simulink model "testFrame_PIControler"  (R2020b)
settings: Solver=FixedStepDiscrete  StartTime=0.0  StopTime=10.0  FixedStep=2e-4  RelTol=1e-3
undefined symbols (not defined in the file): BrkPoints, Down, Ki_dAxis, Ki_qAxis, Kp_dAxis, Kp_qAxis, pwmTableData, Ts, Up
libraries: eePwmGenerator x3, mcbcontrolslib x2
settings Model: DataDictionary=MotorControl.sldd  Creator=unix  LastModifiedBy=unix
settings DebuggingCC: SignalRangeChecking=error  IntegerOverflowMsg=error  ParameterUnderflowMsg=error  IntegerSaturationMsg=error

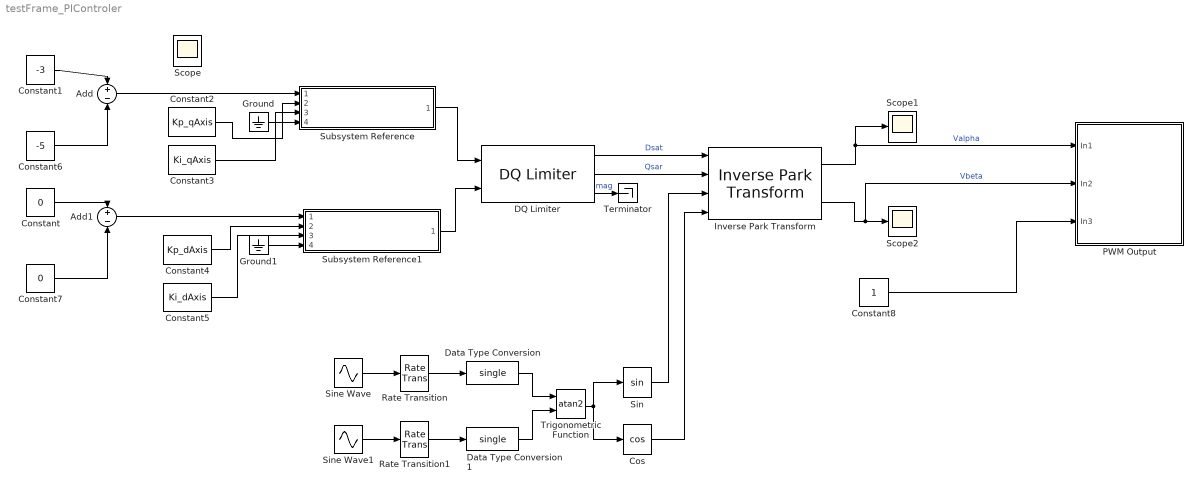
== system testFrame_PIControler ==
  Add : Sum  Inputs=+-
  Add1 : Sum  Inputs=+-
  Constant : Constant  Value=0  OutDataTypeStr=single
  Constant1 : Constant  Value=-3  OutDataTypeStr=single
  Constant2 : Constant  Value=Kp_qAxis  OutDataTypeStr=single
  Constant3 : Constant  Value=Ki_qAxis  OutDataTypeStr=single
  Constant4 : Constant  Value=Kp_dAxis  OutDataTypeStr=single
  Constant5 : Constant  Value=Ki_dAxis  OutDataTypeStr=single
  Constant6 : Constant  Value=-5  OutDataTypeStr=single
  Constant7 : Constant  Value=0  OutDataTypeStr=single
  Constant8 : Constant
  Cos : Trigonometry  Operator=cos
  DQ Limiter : mcbcontrolslib/DQ Limiter  Vmax=d_q_Voltage_Limiter_max
      settings: SourceProductBaseCode=MT
  Data Type Conversion : DataTypeConversion  OutDataTypeStr=single
  Data Type Conversion1 : DataTypeConversion  OutDataTypeStr=single
  Ground : Ground
  Ground1 : Ground
  Inverse Park Transform : mcbcontrolslib/Inverse Park Transform  AxisAlignment=D-axis
  PWM Output : Subsystem
  Rate Transition : RateTransition
  Rate Transition1 : RateTransition
  Scope1 : Scope
  Scope2 : Scope
  Sin : Trigonometry
  Sine Wave : Sin  Amplitude=3  Frequency=60  SampleTime=0
  Sine Wave1 : Sin  Amplitude=3  Frequency=60  Phase=pi/2  SampleTime=0
  Subsystem Reference : Subsystem  ReferencedSubsystem=PID_custom
  Subsystem Reference1 : Subsystem  ReferencedSubsystem=PID_custom
  Terminator : Terminator
  Trigonometric Function : Trigonometry  Operator=atan2
  Scope : Scope
  wires:
  Add/1 -> Subsystem Reference/1
  Add1/1 -> Subsystem Reference1/1
  Constant/1 -> Add1/1
  Constant1/1 -> Add/1
  Ground/1 -> Subsystem Reference/4
  Ground1/1 -> Subsystem Reference1/4
  Constant2/1 -> Subsystem Reference/2
  Constant3/1 -> Subsystem Reference/3
  Constant4/1 -> Subsystem Reference1/2
  Constant5/1 -> Subsystem Reference1/3
  Subsystem Reference/1 -> DQ Limiter/1
  Subsystem Reference1/1 -> DQ Limiter/2
  DQ Limiter/1 -> Inverse Park Transform/1  "Dsat"
  DQ Limiter/2 -> Inverse Park Transform/2  "Qsar"
  DQ Limiter/3 -> Terminator/1  "mag"
  Constant6/1 -> Add/2
  Constant7/1 -> Add1/2
  Sine Wave/1 -> Rate Transition/1
  Sine Wave1/1 -> Rate Transition1/1
  Rate Transition/1 -> Data Type Conversion/1
  Rate Transition1/1 -> Data Type Conversion1/1
  Data Type Conversion/1 -> Trigonometric Function/1
  Data Type Conversion1/1 -> Trigonometric Function/2
  Cos/1 -> Inverse Park Transform/4
  Trigonometric Function/1 -> Sin/1, Cos/1
  Sin/1 -> Inverse Park Transform/3
  Inverse Park Transform/2 -> PWM Output/2(In2), Scope2/1  "Vbeta"
  Inverse Park Transform/1 -> PWM Output/1(In1), Scope1/1  "Valpha"
  Constant8/1 -> PWM Output/3(In3)

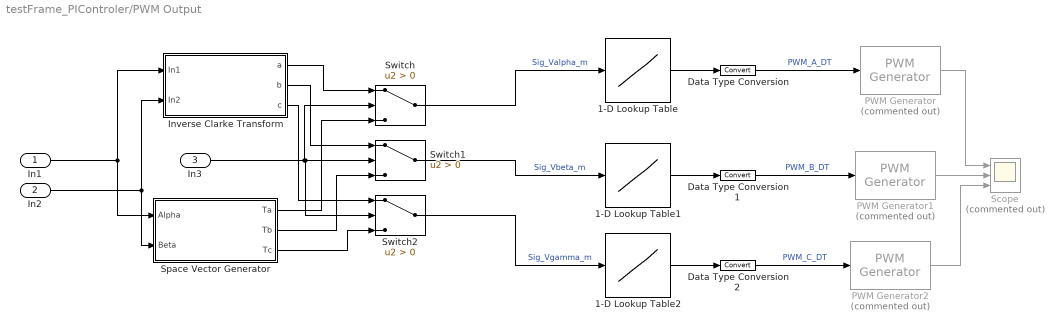
== system testFrame_PIControler/PWM Output ==
  In1 : Inport
  In2 : Inport  Port=2
  In3 : Inport  Port=3
  1-D Lookup Table : Lookup_n-D  NumberOfTableDimensions=1  BreakpointsForDimension1=BrkPoints  Table=pwmTableData  ExtrapMethod=Clip  InternalRulePriority=Speed  OutDataTypeStr=uint16  RndMeth=Simplest  SaturateOnIntegerOverflow=on  InputSameDT=on
  1-D Lookup Table1 : Lookup_n-D  NumberOfTableDimensions=1  BreakpointsForDimension1=BrkPoints  Table=pwmTableData  ExtrapMethod=Clip  InternalRulePriority=Speed  OutDataTypeStr=uint16  RndMeth=Simplest  SaturateOnIntegerOverflow=on  InputSameDT=on
  1-D Lookup Table2 : Lookup_n-D  NumberOfTableDimensions=1  BreakpointsForDimension1=BrkPoints  Table=pwmTableData  ExtrapMethod=Clip  InternalRulePriority=Speed  OutDataTypeStr=uint16  RndMeth=Simplest  SaturateOnIntegerOverflow=on  InputSameDT=on
  Data Type Conversion : DataTypeConversion
  Data Type Conversion1 : DataTypeConversion
  Data Type Conversion2 : DataTypeConversion
  Inverse Clarke Transform : Subsystem  TreatAsAtomicUnit=on  mask(Inverse Clarke Transform){}
      mask help:
      | <p>Compute Inverse Clarke transformation on balanced 2-phase orthogonal inputs into balanced 3-phase outputs.
      | <br><br>
      | The block accepts &alpha;-&beta; axis components and outputs corresponding 3-phase outputs, where phase-a axis is aligned with &alpha;-axis.</p>
      mask Help: eval('mcb.internal.helpview(''inverseclarketransform'')')
      mask Display: mcb.internal.drawIcons('invClarke',1);
  PWM Generator : eePwmGenerator/PWM Generator  Commented=on  CarrCount=Up-Down  Tper=10*Ts  Ts=Ts
  PWM Generator1 : eePwmGenerator/PWM Generator  Commented=on  CarrCount=Up-Down  Tper=10*Ts  Ts=Ts
  PWM Generator2 : eePwmGenerator/PWM Generator  Commented=on  CarrCount=Up-Down  Tper=10*Ts  Ts=Ts
  Scope : Scope  Commented=on  NumInputPorts=3
  Space Vector Generator : Subsystem  TreatAsAtomicUnit=on  mask(Space Vector Generator){}
      mask help:
      | <p>Generate space vector modulation signals from stator reference voltages described by  &alpha;-&beta; components.
      | <br><br>
      | The block accepts V<sub>&alpha;</sub> and V<sub>&beta;</sub> voltages and outputs corresponding space vector modulation voltages.</p>
      mask Help: eval('mcb.internal.helpview(''spacevectorgenerator'')')
      mask Display: mcb.internal.drawIcons('SVPWM',1);
  Switch : Switch  Criteria=u2 > Threshold
  Switch1 : Switch  Criteria=u2 > Threshold
  Switch2 : Switch  Criteria=u2 > Threshold
  wires:
  In2/1 -> Space Vector Generator/2(Beta), Inverse Clarke Transform/2(In2)
  In1/1 -> Space Vector Generator/1(Alpha), Inverse Clarke Transform/1(In1)
  Switch/1 -> 1-D Lookup Table/1  "Sig_Valpha_m"
  1-D Lookup Table/1 -> Data Type Conversion/1
  Switch1/1 -> 1-D Lookup Table1/1  "Sig_Vbeta_m"
  Switch2/1 -> 1-D Lookup Table2/1  "Sig_Vgamma_m"
  PWM Generator/1 -> Scope/1
  1-D Lookup Table2/1 -> Data Type Conversion2/1
  1-D Lookup Table1/1 -> Data Type Conversion1/1
  PWM Generator1/1 -> Scope/2
  PWM Generator2/1 -> Scope/3
  Data Type Conversion/1 -> PWM Generator/1  "PWM_A_DT"
  Data Type Conversion1/1 -> PWM Generator1/1  "PWM_B_DT"
  Data Type Conversion2/1 -> PWM Generator2/1  "PWM_C_DT"
  Space Vector Generator/1(Ta) -> Switch/3
  Space Vector Generator/2(Tb) -> Switch1/3
  Space Vector Generator/3(Tc) -> Switch2/3
  Inverse Clarke Transform/1(a) -> Switch/1
  Inverse Clarke Transform/2(b) -> Switch1/1
  Inverse Clarke Transform/3(c) -> Switch2/1
  In3/1 -> Switch2/2, Switch1/2, Switch/2

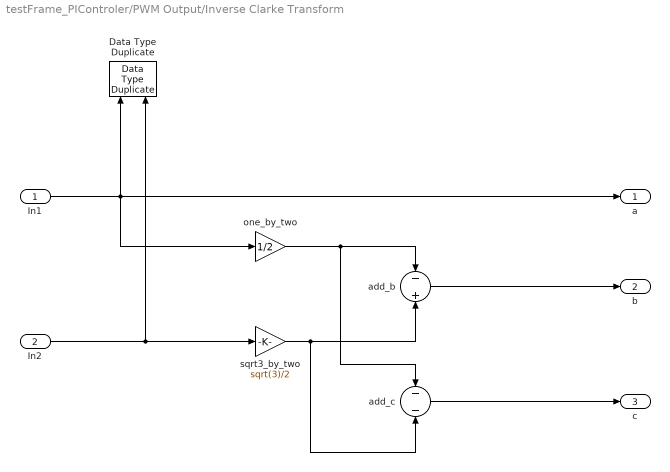
== system testFrame_PIControler/PWM Output/Inverse Clarke Transform ==
  In1 : Inport
  In2 : Inport  Port=2
  Data Type Duplicate : DataTypeDuplicate
  add_b : Sum  Inputs=-+  RndMeth=Simplest  OutDataTypeStr=Inherit: Same as first input
  add_c : Sum  Inputs=--  RndMeth=Simplest  OutDataTypeStr=Inherit: Same as first input
  one_by_two : Gain  Gain=1/2  RndMeth=Simplest  OutDataTypeStr=Inherit: Same as input
  sqrt3_by_two : Gain  Gain=sqrt(3)/2  RndMeth=Simplest  OutDataTypeStr=Inherit: Same as input
  a : Outport  VectorParamsAs1DForOutWhenUnconnected=off
  b : Outport  Port=2  VectorParamsAs1DForOutWhenUnconnected=off
  c : Outport  Port=3  VectorParamsAs1DForOutWhenUnconnected=off
  wires:
  add_c/1 -> c/1
  sqrt3_by_two/1 -> add_c/2, add_b/2
  In1/1 -> one_by_two/1, Data Type Duplicate/1, a/1
  one_by_two/1 -> add_b/1, add_c/1
  In2/1 -> sqrt3_by_two/1, Data Type Duplicate/2
  add_b/1 -> b/1

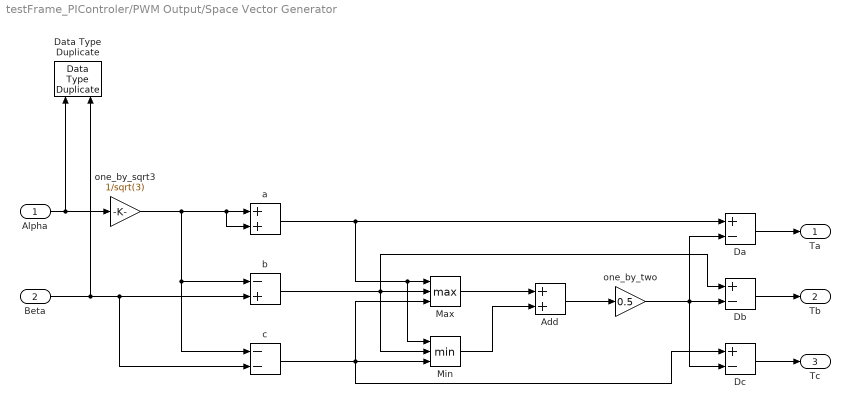
== system testFrame_PIControler/PWM Output/Space Vector Generator ==
  Alpha : Inport
  Beta : Inport  Port=2
  Add : Sum  RndMeth=Simplest  OutDataTypeStr=Inherit: Same as first input
  Da : Sum  Inputs=+-  RndMeth=Simplest  OutDataTypeStr=Inherit: Same as first input
  Data Type Duplicate : DataTypeDuplicate
  Db : Sum  Inputs=+-  RndMeth=Simplest  OutDataTypeStr=Inherit: Same as first input
  Dc : Sum  Inputs=+-  RndMeth=Simplest  OutDataTypeStr=Inherit: Same as first input
  Max : MinMax  Function=max  Inputs=3  RndMeth=Simplest
  Min : MinMax  Inputs=3  RndMeth=Simplest
  a : Sum  RndMeth=Simplest  OutDataTypeStr=Inherit: Same as first input
  b : Sum  Inputs=-+  RndMeth=Simplest  OutDataTypeStr=Inherit: Same as first input
  c : Sum  Inputs=--  RndMeth=Simplest  OutDataTypeStr=Inherit: Same as first input
  one_by_sqrt3 : Gain  Gain=1/sqrt(3)  RndMeth=Simplest  OutDataTypeStr=Inherit: Same as input  ParamDataTypeStr=Inherit: Same as input
  one_by_two : Gain  Gain=0.5  RndMeth=Simplest  OutDataTypeStr=Inherit: Same as input  ParamDataTypeStr=Inherit: Same as input
  Ta : Outport  VectorParamsAs1DForOutWhenUnconnected=off
  Tb : Outport  Port=2  VectorParamsAs1DForOutWhenUnconnected=off
  Tc : Outport  Port=3  VectorParamsAs1DForOutWhenUnconnected=off
  wires:
  Db/1 -> Tb/1
  Dc/1 -> Tc/1
  Da/1 -> Ta/1
  a/1 -> Max/1, Min/1, Da/1
  Max/1 -> Add/1
  one_by_two/1 -> Da/2, Db/2, Dc/2
  Add/1 -> one_by_two/1
  Min/1 -> Add/2
  Alpha/1 -> Data Type Duplicate/1, one_by_sqrt3/1
  one_by_sqrt3/1 -> a/1, a/2, b/1, c/1
  Beta/1 -> c/2, b/2, Data Type Duplicate/2
  b/1 -> Max/2, Min/2, Db/1
  c/1 -> Min/3, Dc/1, Max/3
